simulink model "EoM_test"  (R2023b)
settings: Solver=ode113  StartTime=0.0  StopTime=tf  FixedStep=0.1  RelTol=1e-9  AbsTol=1e-10
undefined symbols (not defined in the file): testCase, w_check
libraries: dyn_lib x3
settings Model: Creator=brent  LastModifiedBy=brent

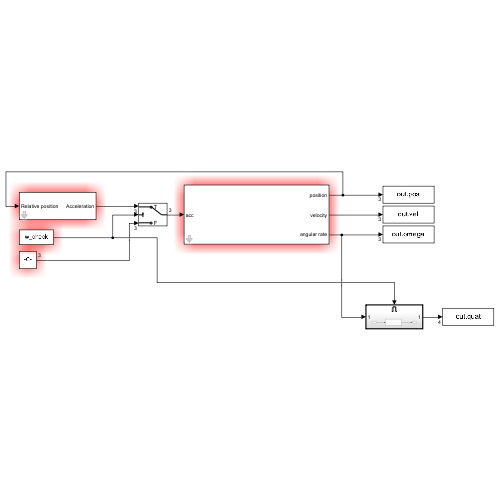
[thumbnail: Simulink's stored preview of the top-level diagram]
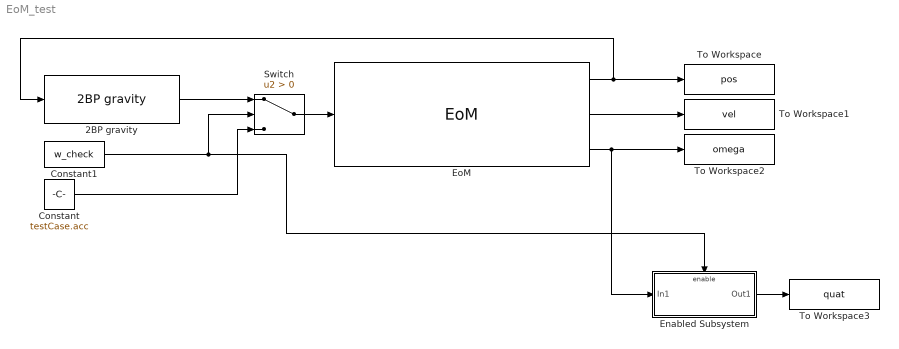
== system EoM_test ==
  2BP gravity : dyn_lib/2BP gravity  mu=testCase.mu
      settings: SourceProductName=Dynamics library
  Constant : Constant  Value=testCase.acc
  Constant1 : Constant  Value=w_check
  Enabled Subsystem : Subsystem  TreatAsAtomicUnit=on
  EoM : dyn_lib/EoM  x0=x0  v0=v0
      settings: SourceProductName=Dynamics library
  Switch : Switch  Criteria=u2 > Threshold  SaturateOnIntegerOverflow=off  InputSameDT=off
  To Workspace : ToWorkspace  VariableName=pos  SampleTime=-1
  To Workspace1 : ToWorkspace  VariableName=vel  SampleTime=-1
  To Workspace2 : ToWorkspace  VariableName=omega  SampleTime=-1
  To Workspace3 : ToWorkspace  VariableName=quat  SampleTime=-1
  wires:
  EoM/1 -> To Workspace/1, 2BP gravity/1
  EoM/2 -> To Workspace1/1
  EoM/3 -> To Workspace2/1, Enabled Subsystem/1(In1)
  Switch/1 -> EoM/1
  2BP gravity/1 -> Switch/1
  Constant/1 -> Switch/3
  Constant1/1 -> Enabled Subsystem/Enable, Switch/2
  Enabled Subsystem/1(Out1) -> To Workspace3/1

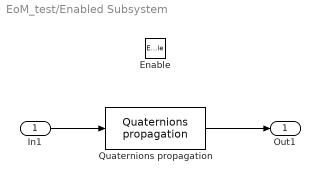
== system EoM_test/Enabled Subsystem ==
  In1 : Inport
  Enable : EnablePort
  Quaternions propagation : dyn_lib/Quaternions propagation  q0=q0
      settings: SourceProductName=Dynamics library
  Out1 : Outport
  wires:
  In1/1 -> Quaternions propagation/1
  Quaternions propagation/1 -> Out1/1
